simulink model "No_Disturbance_Simulation"  (R2024a)
settings: Solver=VariableStepAuto  StartTime=0.0  StopTime=15*3600  RelTol=1e-3
values from neighbouring files (symbols this model uses):
  J0 = (m/12)*(l^2*cos(beta)^2+d^2*sin(beta)^2+w^2)    [Group10_Final_Code_Summer.m]    (also in Group10_Final_Main_Code_Winter.m)
  Kd = 5    [Group10_Final_Code_Summer.m]    (also in Group10_Final_Main_Code_Winter.m)
  Kf = 0.07    [Group10_Final_Code_Summer.m]    (also in Group10_Final_Main_Code_Winter.m)
  Kg = 3000    [Group10_Final_Code_Summer.m]    (also in Group10_Final_Main_Code_Winter.m)
  Kp = 0.318    [Group10_Final_Code_Summer.m]    (also in Group10_Final_Main_Code_Winter.m)
  Kt = 0.07    [Group10_Final_Code_Summer.m]    (also in Group10_Final_Main_Code_Winter.m)
  L = 1e-5    (= 1e-05)    [Group10_Final_Code_Summer.m]    (also in Group10_Final_Main_Code_Winter.m)
  R = 10    [Group10_Final_Code_Summer.m]    (also in Group10_Final_Main_Code_Winter.m)
libraries: slpidlib x1
settings Model: Creator=marin  LastModifiedBy=marin
settings DataIOCC: ExternalInput=[sunTime, sunPosition]  LoadExternalInput=on

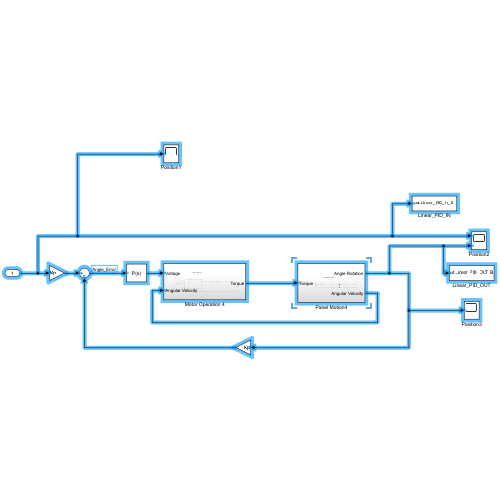
[thumbnail: Simulink's stored preview of the top-level diagram]
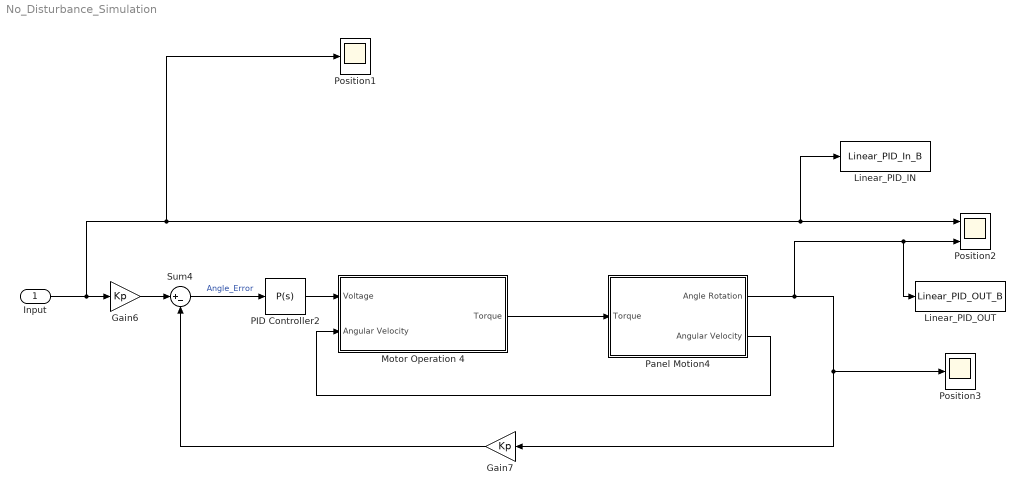
== system No_Disturbance_Simulation ==
  Input : Inport
  Gain6 : Gain  Gain=Kp
  Gain7 : Gain  Gain=Kp
  Linear_PID_IN : ToWorkspace  VariableName=Linear_PID_In_B  SampleTime=-1
  Linear_PID_OUT : ToWorkspace  VariableName=Linear_PID_OUT_B  SampleTime=-1
  Motor Operation 4 : Subsystem
  PID Controller2 : slpidlib/PID Controller  Controller=P  Form=Parallel  TimeDomain=Continuous-time  UseExternalTs=off  SampleTime=-1  IntegratorMethod=Forward Euler  FilterMethod=Forward Euler  ControllerParametersSource=internal  P=4700  I=180  UseKiTs=off  D=0  UseExternalDerivativeSource=off  N=100  UseFilter=on  TunerSelectOption=Transfer Function Based (PID Tuner App)  InitialConditionSource=internal  InitialConditionForIntegrator=0  InitialConditionForFilter=0  DifferentiatorICPrevScaledInput=0  ExternalReset=none  TrackingMode=off  Kt=1  LimitOutput=off  SatLimitsSource=internal  UpperSaturationLimit=inf  LowerSaturationLimit=-inf  LinearizeAsGain=on  AntiWindupMode=none  Kb=1  LimitIntegrator=off  UpperIntegratorSaturationLimit=inf  LowerIntegratorSaturationLimit=-inf  POutMin=[]  POutMax=[]  IOutMin=[]  IOutMax=[]  DOutMin=[]  DOutMax=[]  NOutMin=[]  NOutMax=[]  SumOutMin=[]  SumOutMax=[]  SaturationOutMin=[]  SaturationOutMax=[]  PParamMin=[]  PParamMax=[]  IParamMin=[]  IParamMax=[]  DParamMin=[]  DParamMax=[]  NParamMin=[]  NParamMax=[]  KbParamMin=[]  KbParamMax=[]  KtParamMin=[]  KtParamMax=[]  KbOutMin=[]  KbOutMax=[]  KtOutMin=[]  KtOutMax=[]  IntegratorOutMin=[]  IntegratorOutMax=[]  FilterOutMin=[]  FilterOutMax=[]  SumI1OutMin=[]  SumI1OutMax=[]  SumI2OutMin=[]  SumI2OutMax=[]  SumI3OutMin=[]  SumI3OutMax=[]  SumI4OutMin=[]  SumI4OutMax=[]  SumDOutMin=[]  SumDOutMax=[]  DifferentiatorOutMin=[]  DifferentiatorOutMax=[]  FilterDiffOutCoefMin=[]  FilterDiffOutCoefMax=[]  ReciprocalOutMin=[]  ReciprocalOutMax=[]  SumDenOutMin=[]  SumDenOutMax=[]  SumNumOutMin=[]  SumNumOutMax=[]  DivideOutMin=[]  DivideOutMax=[]  UdiffTsProdOutMin=[]  UdiffTsProdOutMax=[]  NTsProdOutMin=[]  NTsProdOutMax=[]  UintegralTsProdOutMin=[]  UintegralTsProdOutMax=[]  UngainTsProdOutMin=[]  UngainTsProdOutMax=[]  ClampingZeroOutDataTypeStr=Inherit: Inherit via back propagation  ClampingZeroOutMin=[]  ClampingZeroOutMax=[]  FilterDenConstantOutDataTypeStr=Inherit: Inherit via back propagation  FilterDenConstantOutMin=[]  FilterDenConstantOutMax=[]  PCopyOutDataTypeStr=Inherit: Inherit via back propagation  PCopyOutMin=[]  PCopyOutMax=[]  NCopyOutDataTypeStr=Inherit: Inherit via back propagation  NCopyOutMin=[]  NCopyOutMax=[]  IntegratorContinuousStateAttributes=''  IntegratorStateMustResolveToSignalObject=off  IntegratorRTWStateStorageClass=Auto  FilterContinuousStateAttributes=''  FilterStateMustResolveToSignalObject=off  FilterRTWStateStorageClass=Auto  ParallelPVariant=InternalParameters  IdealPVariant=Disabled  IVariant=Disabled  DVariant=Disabled  IntegratorVariant=Disabled  SatVariant=Disabled  AWVariant=Disabled  PCopyVariant=Disabled  TRVariant=Disabled  FdbkBlocksVariant=Forward  IdealPFdbkVariant=Disabled  SatFdbkVariant=Disabled  DerivativeFilterVariant=Disabled  NVariant=Disabled  NCopyVariant=Disabled_SignalSpec  FilterICVariant=Disabled  IntegratorICVariant=Disabled  ExternalResetVariant=Disabled  TRSumVariant=Passthrough  SumFdbkVariant=Disabled  SumVariant=Passthrough_P  TsampFilterVariant=InternalTs  TsampNgainVariant=Passthrough  TsampIntegralVariant=Disabled_SignalSpec  ExternalSaturationOutDataTypeStr=Inherit: Same as second input  DerivativeSourceVariant=Disabled
  Panel Motion4 : Subsystem
  Position1 : Scope
  Position2 : Scope  NumInputPorts=2
  Position3 : Scope
  Sum4 : Sum  Inputs=|+-
  wires:
  Panel Motion4/2(Angular Velocity) -> Motor Operation 4/2(Angular Velocity)
  PID Controller2/1 -> Motor Operation 4/1(Voltage)
  Motor Operation 4/1(Torque) -> Panel Motion4/1(Torque)
  Sum4/1 -> PID Controller2/1  "Angle_Error"
  Panel Motion4/1(Angle Rotation) -> Linear_PID_OUT/1, Position2/2, Position3/1, Gain7/1
  Gain7/1 -> Sum4/2
  Input/1 -> Gain6/1, Position1/1, Linear_PID_IN/1, Position2/1
  Gain6/1 -> Sum4/1

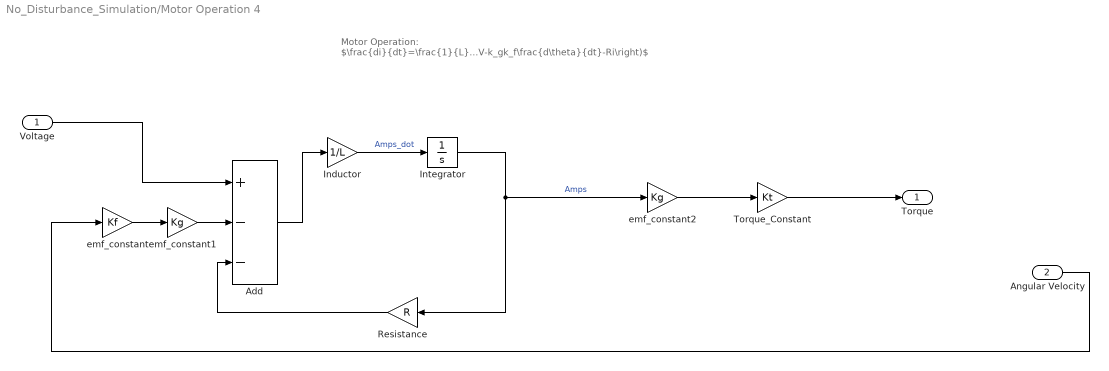
== system No_Disturbance_Simulation/Motor Operation 4 ==
  note: Motor Operation:
      | $\frac{di}{dt}=\frac{1}{L}\left(V-k_gk_f\frac{d\theta}{dt}-Ri\right)$
  Voltage : Inport
  Angular Velocity : Inport  Port=2
  Add : Sum  Inputs=+--
  Inductor : Gain  Gain=1/L
  Integrator : Integrator
  Resistance : Gain  Gain=R
  Torque_Constant : Gain  Gain=Kt
  emf_constant : Gain  Gain=Kf
  emf_constant1 : Gain  Gain=Kg
  emf_constant2 : Gain  Gain=Kg
  Torque : Outport
  wires:
  emf_constant2/1 -> Torque_Constant/1
  emf_constant1/1 -> Add/2
  Torque_Constant/1 -> Torque/1
  Integrator/1 -> emf_constant2/1, Resistance/1  "Amps"
  Voltage/1 -> Add/1
  Angular Velocity/1 -> emf_constant/1
  Inductor/1 -> Integrator/1  "Amps_dot"
  Add/1 -> Inductor/1
  Resistance/1 -> Add/3
  emf_constant/1 -> emf_constant1/1

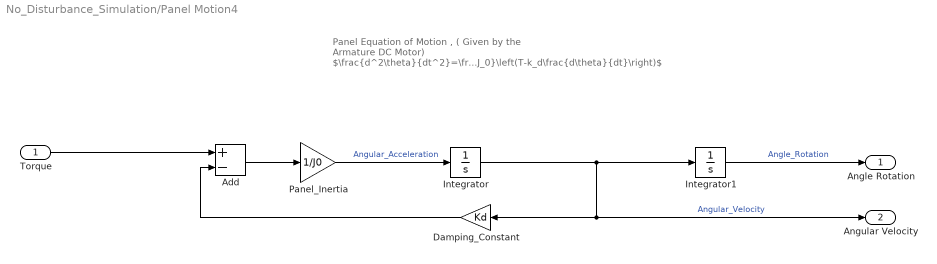
== system No_Disturbance_Simulation/Panel Motion4 ==
  note: Panel Equation of Motion ,
      | ( Given by the Armature DC Motor)
      | $\frac{d^2\theta}{dt^2}=\frac{1}{J_0}\left(T-k_d\frac{d\theta}{dt}\right)$
  Torque : Inport
  Add : Sum  Inputs=+-
  Damping_Constant : Gain  Gain=Kd
  Integrator : Integrator
  Integrator1 : Integrator
  Panel_Inertia : Gain  Gain=1/J0
  Angle Rotation : Outport
  Angular Velocity : Outport  Port=2
  wires:
  Torque/1 -> Add/1
  Integrator/1 -> Integrator1/1, Damping_Constant/1, Angular Velocity/1  "Angular_Velocity"
  Damping_Constant/1 -> Add/2
  Add/1 -> Panel_Inertia/1
  Panel_Inertia/1 -> Integrator/1  "Angular_Acceleration"
  Integrator1/1 -> Angle Rotation/1  "Angle_Rotation"
